simulink model "PID_my"  (Simulink 8.7)
settings: Solver=ode4  StartTime=0.0  StopTime=40  RelTol=1e-3
settings Model: Creator=yyy  LastModifiedBy=yyy
settings DataIOCC: SignalLoggingSaveFormat=ModelDataLogs
settings OptimizationCC: InitFltsAndDblsToZero=on
settings DebuggingCC: SaveWithParameterizedLinksMsg=none  SignalResolutionControl=TryResolveAllWithWarning  SolverPrmCheckMsg=warning  MultiTaskDSMMsg=warning  MultiTaskCondExecSysMsg=none  FcnCallInpInsideContextMsg=UseLocalSettings
settings GRTTargetCC: TargetFcnLib=ansi_tfl_tmw.mat  GeneratePreprocessorConditionals=Use local settings  CombineOutputUpdateFcns=off  GRTInterface=on

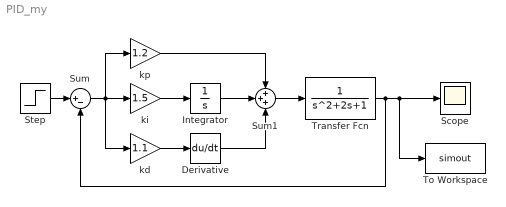
== system PID_my ==
  Derivative : Derivative
  Integrator : Integrator
  Scope : Scope
  Step : Step  SampleTime=0
  Sum : Sum  Inputs=|+-  SaturateOnIntegerOverflow=on  InputSameDT=on  OutDataTypeStr=Inherit: Same as first input
  Sum1 : Sum  Inputs=+++  SaturateOnIntegerOverflow=on  InputSameDT=on  OutDataTypeStr=Inherit: Same as first input
  To Workspace : ToWorkspace  VariableName=simout  SaveFormat=Structure  SampleTime=-1
  Transfer Fcn : TransferFcn  Numerator=1
  "kd " : Gain  Gain=1.1
  ki : Gain  Gain=1.5
  kp : Gain  Gain=1.2
  wires:
  Step/1 -> Sum/1
  Sum/1 -> "kd "/1, kp/1, ki/1
  ki/1 -> Integrator/1
  kp/1 -> Sum1/1
  Integrator/1 -> Sum1/2
  Sum1/1 -> Transfer Fcn/1
  Transfer Fcn/1 -> Scope/1, To Workspace/1, Sum/2
  "kd "/1 -> Derivative/1
  Derivative/1 -> Sum1/3
